simulink model "neww"  (R2023a)
settings: Solver=VariableStepAuto  StartTime=0.0  StopTime=0.5  RelTol=1e-3
libraries: spsMosfetLib x14, spsSeriesRLCBranchLib x13, simulink x6, spsDiodeLib x6, spsCurrentMeasurementLib x4, spsVoltageMeasurementLib x4, spsDCVoltageSourceLib x1, slpidlib x1, spsPVArrayLib x1, spsPWMGeneratorDCDCLib x1, spspowerguiLib x1
settings Model: Creator=91790  LastModifiedBy=USER
settings DataIOCC: ReturnWorkspaceOutputs=off
settings RTWCC: GPUComputeCapability=5.0

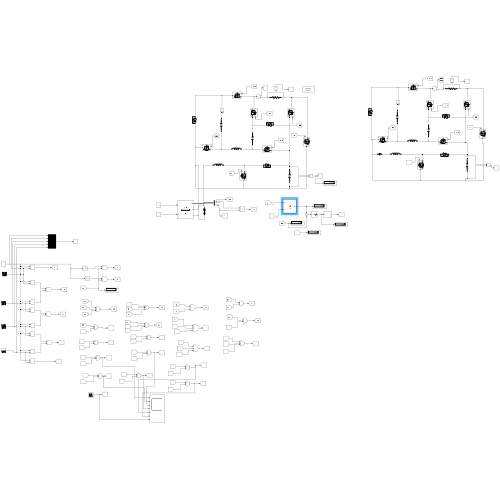
[thumbnail: Simulink's stored preview of the top-level diagram]
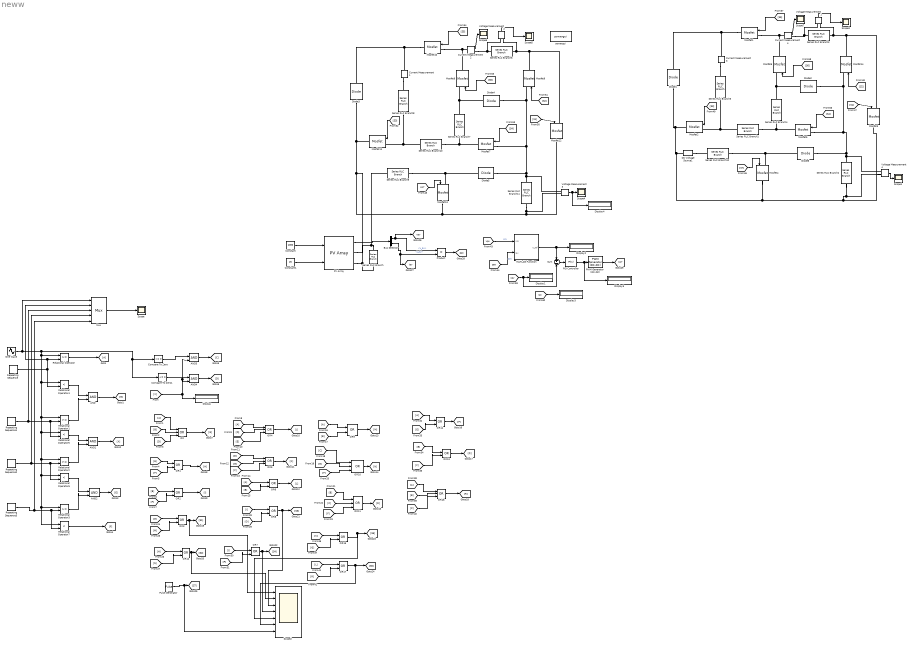
== system neww ==
  AND{,1..4} (5 alike) : Logic  IconShape=distinctive  AllPortsSameDT=off  OutDataTypeStr=boolean
  Bus Selector : BusSelector  OutputSignals=V_PV,I_PV
  Compare To Zero : simulink/Logic and Bit Operations/Compare To Zero  relop=>=  OutDataTypeStr=boolean
  Compare To Zero1 : simulink/Logic and Bit Operations/Compare To Zero  relop=<=  OutDataTypeStr=boolean
  Constant : Constant  Value=1000
  Constant1 : Constant  Value=25
  Current Measurement{1..4} (4 alike) : spsCurrentMeasurementLib/Current Measurement  PhasorSimulation=off  OutputType=Complex  PSBequivalent=0
  DC Voltage Source1 : spsDCVoltageSourceLib/DC Voltage Source  Amplitude=8  Measurements=None
  Diode{1..6} (6 alike) : spsDiodeLib/Diode  Ron=0.001  Lon=0  Vf=0.8  IC=0  UseSnubber=0  Rs=500  Cs=250e-9  Measurements=off
  Display{,1..5} (6 alike) : Display
  From{1,8,14,16,32,38} (6 alike) : From
  Goto : Goto
  MATLAB Function : MATLAB Function  TreatAsAtomicUnit=on  SystemSampleTime=1e-4
  Mosfet{1..14} (14 alike) : spsMosfetLib/Mosfet  Ron=0.1  Lon=0  Rd=0.01  Vfd=0  IC=0  Rs=1e5  Cs=inf  Measurements=off
  Mux : Mux  Inputs=5
  OR{,4..5,10..11,16} (6 alike) : Logic  Operator=OR  Inputs=3  IconShape=distinctive  AllPortsSameDT=off  OutDataTypeStr=boolean
  OR{1..3,6..9,12..15,17} (12 alike) : Logic  Operator=OR  IconShape=distinctive  AllPortsSameDT=off  OutDataTypeStr=boolean
  PID Controller : slpidlib/PID Controller  Controller=PI  Form=Parallel  TimeDomain=Continuous-time  UseExternalTs=off  SampleTime=-1  IntegratorMethod=Forward Euler  FilterMethod=Forward Euler  ControllerParametersSource=internal  P=0  I=-15  UseKiTs=off  D=0  N=100  UseFilter=on  TunerSelectOption=Transfer Function Based (PID Tuner App)  InitialConditionSource=internal  InitialConditionForIntegrator=0.5  InitialConditionForFilter=0  DifferentiatorICPrevScaledInput=0  ExternalReset=none  TrackingMode=off  Kt=1  LimitOutput=on  SatLimitsSource=internal  UpperSaturationLimit=0.95  LowerSaturationLimit=0.05  LinearizeAsGain=off  AntiWindupMode=none  Kb=1  LimitIntegrator=off  UpperIntegratorSaturationLimit=inf  LowerIntegratorSaturationLimit=-inf  POutMin=[]  POutMax=[]  IOutMin=[]  IOutMax=[]  DOutMin=[]  DOutMax=[]  NOutMin=[]  NOutMax=[]  SumOutMin=[]  SumOutMax=[]  SaturationOutMin=[]  SaturationOutMax=[]  PParamMin=[]  PParamMax=[]  IParamMin=[]  IParamMax=[]  DParamMin=[]  DParamMax=[]  NParamMin=[]  NParamMax=[]  KbParamMin=[]  KbParamMax=[]  KtParamMin=[]  KtParamMax=[]  KbOutMin=[]  KbOutMax=[]  KtOutMin=[]  KtOutMax=[]  IntegratorOutMin=[]  IntegratorOutMax=[]  FilterOutMin=[]  FilterOutMax=[]  SumI1OutMin=[]  SumI1OutMax=[]  SumI2OutMin=[]  SumI2OutMax=[]  SumI3OutMin=[]  SumI3OutMax=[]  SumI4OutMin=[]  SumI4OutMax=[]  SumDOutMin=[]  SumDOutMax=[]  DifferentiatorOutMin=[]  DifferentiatorOutMax=[]  FilterDiffOutCoefMin=[]  FilterDiffOutCoefMax=[]  ReciprocalOutMin=[]  ReciprocalOutMax=[]  SumDenOutMin=[]  SumDenOutMax=[]  SumNumOutMin=[]  SumNumOutMax=[]  DivideOutMin=[]  DivideOutMax=[]  UdiffTsProdOutMin=[]  UdiffTsProdOutMax=[]  NTsProdOutMin=[]  NTsProdOutMax=[]  UintegralTsProdOutMin=[]  UintegralTsProdOutMax=[]  UngainTsProdOutMin=[]  UngainTsProdOutMax=[]  ClampingZeroOutDataTypeStr=Inherit: Inherit via back propagation  ClampingZeroOutMin=[]  ClampingZeroOutMax=[]  FilterDenConstantOutDataTypeStr=Inherit: Inherit via back propagation  FilterDenConstantOutMin=[]  FilterDenConstantOutMax=[]  PCopyOutDataTypeStr=Inherit: Inherit via back propagation  PCopyOutMin=[]  PCopyOutMax=[]  NCopyOutDataTypeStr=Inherit: Inherit via back propagation  NCopyOutMin=[]  NCopyOutMax=[]  IntegratorContinuousStateAttributes=''  IntegratorStateMustResolveToSignalObject=off  IntegratorRTWStateStorageClass=Auto  FilterContinuousStateAttributes=''  FilterStateMustResolveToSignalObject=off  FilterRTWStateStorageClass=Auto  ParallelPVariant=InternalParameters  IdealPVariant=Disabled  IVariant=InternalParameters  DVariant=Disabled  IntegratorVariant=Continuous  SatVariant=Enabled  AWVariant=Passthrough  PCopyVariant=Disabled  TRVariant=Disabled  FdbkBlocksVariant=Forward  IdealPFdbkVariant=Disabled  SatFdbkVariant=Disabled  DerivativeFilterVariant=Disabled  NVariant=Disabled  NCopyVariant=Disabled_SignalSpec  FilterICVariant=Disabled  IntegratorICVariant=InternalICs  ExternalResetVariant=Disabled  TRSumVariant=Passthrough  SumFdbkVariant=Disabled  SumVariant=Sum_PI  TsampFilterVariant=InternalTs  TsampNgainVariant=Passthrough  TsampIntegralVariant=Disabled_SignalSpec  ExternalSaturationOutDataTypeStr=Inherit: Same as second input
  PV Array : spsPVArrayLib/PV Array  Npar=1  Nser=1  PlotType=array @ 1000 W/m2 & specified temperatures  S_vec="[ 1000  500  100 ]"  Temp_C_vec="[ 45 25  ]"  ModuleName=User-defined  PlotWhenSelected=off  Pm=74.8334  Ncell=36  Voc=21.89  Isc=4.48  Vm=17.86  Im=4.19  beta_Voc_pc=-0.36099  alpha_Isc_pc=0.102  beta_Voc=-0.079021  alpha_Isc=0.0045696  IL=4.485  I0=1.6678e-10  nI=0.98621  Rsh=286.612  Rs=0.317  RobustModel=off  RobustCellTemperature=313.3991  BAL=on  Tc=1e-6  Tfilter=5e-5
  PWM Generator (DC-DC) : spsPWMGeneratorDCDCLib/PWM Generator (DC-DC)  Fsw=2500  Ts=0
  Product : Product
  Pulse Generator : DiscretePulseGenerator  PulseType=Time based  Period=1/21000  PulseWidth=75
  Relational Operator{,1..3} (4 alike) : RelationalOperator  OutDataTypeStr=boolean  RndMeth=Simplest  InputSameDT=off
  Relational Operator{4..7} (4 alike) : RelationalOperator  Operator=<  OutDataTypeStr=boolean  RndMeth=Simplest  InputSameDT=off
  Repeating Sequence : simulink/Sources/Repeating Sequence  rep_seq_t=[0 1/4 1/2]/2500  rep_seq_y=[1 0.5 1]
  Repeating Sequence1 : simulink/Sources/Repeating Sequence  rep_seq_t=[0 1/4 1/2]/2500  rep_seq_y=[0.5 0 0.5]
  Repeating Sequence2 : simulink/Sources/Repeating Sequence  rep_seq_t=[0 1/4 1/2]/2500  rep_seq_y=[0 -0.5 0]
  Repeating Sequence3 : simulink/Sources/Repeating Sequence  rep_seq_t=[0 1/4 1/2]/2500  rep_seq_y=[-0.5 -1 -0.5]
  Scope{,1,3..7} (7 alike) : Scope
  Scope2 : Scope  NumInputPorts=7
  Series RLC Branch : spsSeriesRLCBranchLib/Series RLC Branch  LConnTagsString=__new0  RConnTagsString=__new0  BranchType=RC  Resistance=0.11e-4  Inductance=1e-3  SetiL0=off  InitialCurrent=0  Capacitance=1000e-6  Setx0=off  InitialVoltage=0  Measurements=None
  Series RLC Branch1 : spsSeriesRLCBranchLib/Series RLC Branch  LConnTagsString=__new0  RConnTagsString=__new0  BranchType=L  Resistance=100  Inductance=1e-3  SetiL0=off  InitialCurrent=0  Capacitance=1e-6  Setx0=off  InitialVoltage=0  Measurements=Branch voltage and current
  Series RLC Branch10 : spsSeriesRLCBranchLib/Series RLC Branch  LConnTagsString=__new0  RConnTagsString=__new0  BranchType=L  Resistance=100  Inductance=1e-3  SetiL0=off  InitialCurrent=0  Capacitance=1e-6  Setx0=off  InitialVoltage=0  Measurements=Branch voltage and current
  Series RLC Branch11 : spsSeriesRLCBranchLib/Series RLC Branch  LConnTagsString=__new0  RConnTagsString=__new0  BranchType=C  Resistance=100  Inductance=1e-3  SetiL0=off  InitialCurrent=0  Capacitance=4700e-6  Setx0=off  InitialVoltage=0  Measurements=None
  Series RLC Branch12 : spsSeriesRLCBranchLib/Series RLC Branch  LConnTagsString=__new0  RConnTagsString=__new0  BranchType=L  Resistance=100  Inductance=1e-3  SetiL0=off  InitialCurrent=0  Capacitance=1e-6  Setx0=off  InitialVoltage=0  Measurements=None
  Series RLC Branch{2,4..5,7..8} (5 alike) : spsSeriesRLCBranchLib/Series RLC Branch  LConnTagsString=__new0  RConnTagsString=__new0  BranchType=C  Resistance=100  Inductance=1e-3  SetiL0=off  InitialCurrent=0  Capacitance=2200e-6  Setx0=off  InitialVoltage=0  Measurements=None
  Series RLC Branch3 : spsSeriesRLCBranchLib/Series RLC Branch  LConnTagsString=__new0  RConnTagsString=__new0  BranchType=R  Resistance=100  Inductance=5e-3  SetiL0=off  InitialCurrent=0  Capacitance=1e-6  Setx0=off  InitialVoltage=0  Measurements=None
  Series RLC Branch6 : spsSeriesRLCBranchLib/Series RLC Branch  LConnTagsString=__new0  RConnTagsString=__new0  BranchType=R  Resistance=100  Inductance=5e-3  SetiL0=off  InitialCurrent=0  Capacitance=1e-6  Setx0=off  InitialVoltage=0  Measurements=None
  Series RLC Branch9 : spsSeriesRLCBranchLib/Series RLC Branch  LConnTagsString=__new0  RConnTagsString=__new0  BranchType=L  Resistance=100  Inductance=1e-3  SetiL0=off  InitialCurrent=0  Capacitance=1e-6  Setx0=off  InitialVoltage=0  Measurements=None
  Sine Wave : Sin  Amplitude=0.98  Frequency=2*pi*50  SampleTime=0
  Sum : Sum  Inputs=+-
  Voltage Measurement{1..4} (4 alike) : spsVoltageMeasurementLib/Voltage Measurement  PhasorSimulation=off  OutputType=Complex  PSBequivalent=0
  powergui : spspowerguiLib/powergui  Priority=1  SimulationMode=Discrete  SampleTime=5e-6  frequency=60  Iterations=50  frequencyindice=0  Pbase=100e6  ErrMax=1e-4  UnitsV=kV  UnitsW=MW  buscounter=0  FunctionMessages=off  echomessages=off  EnableUseOfTLC=off  CurrentSourceSwitches=off  DisableSnubberDevices=off  DisableRonSwitches=off  DisableVfSwitches=off  DisplayEquations=off  AutomaticDiscreteSolvers=off  SolverType=Tustin/Backward Euler (TBE)  Interpol=off  ExternalGateDelay=off  methode=off  Ts=100  x0status=blocks  SPID=on  SwTol=0  HookPort=off  NonlinearTolerance=1e-4  nMaxIteration=100  ContinueOnMaxIteration=off  RestoreLinks=warning  ResistiveCurrentMeasurement=off  Frange=[0:2:500]  Ylog=off  Xlog=on  ShowGrid=off  save=off  variable=ZData  structure=0  ZoomFFT=off  StartTime=0.0  cycles=1  DisplayStyle=1  fundamental=60  FreqAxis=off  MaxFrequency=1000  frequencyindicesteady=1  RmsSteady=1  display=off
  tag scope: ipv=global, ppv=global, ss7=global, vpv=global
  wires:
  Repeating Sequence/1 -> Relational Operator4/2, Mux/2, Relational Operator/2
  Repeating Sequence1/1 -> Relational Operator5/2, Relational Operator1/2, Mux/3
  Repeating Sequence2/1 -> Relational Operator2/2, Relational Operator6/2, Mux/4
  Repeating Sequence3/1 -> Relational Operator3/2, Relational Operator7/2, Mux/5
  Relational Operator4/1 -> AND/1
  Relational Operator1/1 -> AND/2
  Relational Operator5/1 -> AND1/1
  Relational Operator2/1 -> AND1/2
  Relational Operator6/1 -> AND2/1
  Relational Operator3/1 -> AND2/2
  Compare To Zero/1 -> AND3/1
  Compare To Zero1/1 -> AND4/1
  [X] -> AND4/2, AND3/2, Display/1
  AND3/1 -> [C]
  AND4/1 -> [D]
  From1/1 -> OR/1
  [B] -> OR/2
  [D] -> OR/3
  [E] -> OR1/1
  [F] -> OR1/2
  [B] -> OR2/1
  [F] -> OR2/2
  OR/1 -> [G]
  OR1/1 -> [H]
  OR2/1 -> [I]
  OR4/1 -> [J]
  From8/1 -> OR4/1
  [D] -> OR4/2
  [E] -> OR4/3
  [D] -> OR5/1
  [E] -> OR5/2
  [F] -> OR5/3
  From14/1 -> OR6/1
  [B] -> OR6/2
  OR5/1 -> [K]
  OR6/1 -> [L]
  OR9/1 -> [M]
  [C] -> OR10/1
  [F] -> OR10/3
  [F] -> OR11/3
  OR10/1 -> [N]
  [E] -> OR10/2
  OR11/1 -> [O]
  [C] -> OR11/2
  [B] -> OR11/1
  [G] -> OR3/1
  [M] -> OR3/2
  [N] -> OR12/2
  [H] -> OR12/1
  [J] -> OR7/1
  [P] -> OR7/2
  [O] -> OR8/2
  [I] -> OR8/1
  [F] -> OR13/2
  [E] -> OR14/2
  From32/1 -> OR14/1
  [E] -> OR13/1
  OR13/1 -> [Q]
  OR14/1 -> [P]
  [Q] -> OR15/2
  [K] -> OR15/1
  From38/1 -> OR16/1
  OR16/1 -> [R]
  [B] -> OR16/2
  [C] -> OR16/3
  Relational Operator/1 -> Goto/1
  AND/1 -> [B]
  AND1/1 -> [X]
  AND2/1 -> [E]
  Relational Operator7/1 -> [F]
  Sine Wave/1 -> Mux/1, Compare To Zero1/1, Compare To Zero/1, Relational Operator/1, Relational Operator4/1, Relational Operator1/1, Relational Operator5/1, Relational Operator2/1, Relational Operator6/1, Relational Operator3/1, Relational Operator7/1
  Mux/1 -> Scope/1
  OR3/1 -> Scope2/1, [S1]
  OR12/1 -> Scope2/2, [S2]
  OR8/1 -> Scope2/3, [S3]
  OR7/1 -> Scope2/4, [S4]
  [L] -> OR17/1
  [R] -> OR17/2
  OR15/1 -> Scope2/5, [S5]
  OR17/1 -> Scope2/6, [S6]
  Pulse Generator/1 -> Scope2/7, [S7]
  From16/1 -> OR9/1
  [B] -> OR9/2
  Voltage Measurement3/1 -> Display4/1, Scope4/1
  [ss7] -> Mosfet13/1
  Voltage Measurement2/1 -> Scope5/1
  [S2] -> Mosfet9/1
  [S1] -> Mosfet12/1
  [S6] -> Mosfet8/1
  [S5] -> Mosfet10/1
  [S4] -> Mosfet7/1
  [S3] -> Mosfet11/1
  Current Measurement2/1 -> Scope6/1
  Constant1/1 -> PV Array/2
  Constant/1 -> PV Array/1
  Bus Selector/2 -> [ipv], Product/2  "<I_PV>"
  Bus Selector/1 -> Product/1, [vpv]  "<V_PV>"
  PV Array/1 -> Bus Selector/1
  [ppv] -> MATLAB Function/2(ipv)  "ppv"
  Product/1 -> [ppv]
  [vpv] -> MATLAB Function/1(vpv)  "vpv"
  MATLAB Function/1(V_ref) -> Sum/1, Display2/1
  Current Measurement4/1 -> Scope7/1
  [S3] -> Mosfet2/1
  [S4] -> Mosfet5/1
  [S5] -> Mosfet1/1
  [S6] -> Mosfet6/1
  [S1] -> Mosfet3/1
  [S2] -> Mosfet14/1
  Voltage Measurement1/1 -> Scope3/1
  [S7] -> Mosfet4/1
  Voltage Measurement4/1 -> Scope1/1
  [vpv] -> Sum/2, Display1/1
  [ipv] -> Display3/1
  Sum/1 -> PID Controller/1
  PID Controller/1 -> Display5/1, PWM Generator (DC-DC)/1
  PWM Generator (DC-DC)/1 -> [ss7]
  connections:
  Diode3/RConn1 -- Mosfet13/RConn1 -- Series RLC Branch11/RConn1 -- Voltage Measurement3/LConn2 -- Mosfet12/RConn1 -- PV Array/RConn2 -- Series RLC Branch/RConn1 -- Mosfet11/RConn1
  Voltage Measurement2/LConn1 -- Series RLC Branch6/RConn1 -- Mosfet12/LConn1 -- Mosfet9/RConn1
  Mosfet10/RConn1 -- Diode3/LConn1 -- Current Measurement1/LConn1
  Mosfet10/LConn1 -- Current Measurement2/LConn1 -- Mosfet8/RConn1
  Mosfet11/LConn1 -- Series RLC Branch8/LConn1 -- Series RLC Branch10/LConn1
  Diode4/LConn1 -- Mosfet7/LConn1 -- Voltage Measurement3/LConn1 -- Series RLC Branch11/LConn1 -- Diode5/RConn1 -- Mosfet9/LConn1
  Series RLC Branch7/RConn1 -- Mosfet7/RConn1 -- Series RLC Branch10/RConn1
  Diode4/RConn1 -- Series RLC Branch7/LConn1 -- Mosfet8/LConn1
  Series RLC Branch9/RConn1 -- Mosfet13/LConn1 -- Diode5/LConn1
  Current Measurement1/RConn1 -- Series RLC Branch8/RConn1
  Series RLC Branch6/LConn1 -- Voltage Measurement2/LConn2 -- Current Measurement2/RConn1
  Mosfet3/RConn1 -- Voltage Measurement4/LConn2 -- Series RLC Branch2/RConn1 -- Diode1/RConn1 -- Mosfet2/RConn1 -- DC Voltage Source1/LConn1 -- Mosfet4/RConn1
  Voltage Measurement1/LConn1 -- Mosfet14/RConn1 -- Mosfet3/LConn1 -- Series RLC Branch3/RConn1
  Mosfet1/RConn1 -- Current Measurement3/LConn1 -- Diode1/LConn1
  Mosfet1/LConn1 -- Mosfet6/RConn1 -- Current Measurement4/LConn1
  Mosfet2/LConn1 -- Series RLC Branch1/LConn1 -- Series RLC Branch5/LConn1
  Diode2/LConn1 -- Mosfet14/LConn1 -- Diode6/RConn1 -- Series RLC Branch2/LConn1 -- Voltage Measurement4/LConn1 -- Mosfet5/LConn1
  Series RLC Branch4/RConn1 -- Series RLC Branch1/RConn1 -- Mosfet5/RConn1
  Diode2/RConn1 -- Mosfet6/LConn1 -- Series RLC Branch4/LConn1
  Series RLC Branch12/RConn1 -- Diode6/LConn1 -- Mosfet4/LConn1
  Series RLC Branch3/LConn1 -- Current Measurement4/RConn1 -- Voltage Measurement1/LConn2
  Current Measurement3/RConn1 -- Series RLC Branch5/RConn1
  DC Voltage Source1/RConn1 -- Series RLC Branch12/LConn1
  Series RLC Branch/LConn1 -- PV Array/RConn1 -- Series RLC Branch9/LConn1

== matlab function neww/MATLAB Function ==
  data: vpv input; V_ref output; ipv input
function V_ref = IC_Vref(vpv, ipv)
% Incremental Conductance (IC) MPPT Algorithm for V_ref control
%
% This function determines the new reference voltage (V_ref) for the PV
% system based on the Incremental Conductance rule: dI/dV = -I/V at MPP.
%
% Inputs:
%   vpv - Current PV Voltage (V)
%   ipv - Current PV Current (I)
%
% Output:
%   V_ref - New reference voltage (V_ref)

% --- Persistent variables to remember state between calls ---
persistent v_pre i_pre V_ref_pre;
% --- Define Panel Limits and Step Size ---
persistent V_ref_max V_ref_min del_V;

% --- Step size for voltage perturbation ---
del_V = 0.05; % Perturb by a small voltage step (e.g., 0.05 Volts)

% --- Initialization (runs only once) ---
if isempty(V_ref_pre)
    % Initial values based on your panel's datasheet (Vmp)
    v_pre = 17.19;     
    i_pre = 74 / 17.19; % Initial current estimate
    V_ref_pre = 17.19; % Start at Vmp
    
    % --- SET LIMITS HERE ---
    V_ref_max = 21.19; % Open Circuit Voltage (Voc)
    V_ref_min = 5.0;   % A safe minimum limit
end

% --- Calculate Changes (Increments) ---
Delta_V = vpv - v_pre;
Delta_I = ipv - i_pre;

% --- Core IC Decision Logic ---
V_ref = V_ref_pre; % Initialize V_ref to the previous value (No change)

% Case 1: Change in Voltage is ZERO (Delta_V = 0)
% This happens if the system is holding steady or if the PI controller is very stiff.
if (Delta_V == 0)
    % Check if power is increasing (I increases) or decreasing (I decreases)
    if (Delta_I > 0)
        % V is constant, I is increasing -> Still increasing power, continue
        V_ref = V_ref_pre + del_V;
    elseif (Delta_I < 0)
        % V is constant, I is decreasing -> Power dropping, reverse
        V_ref = V_ref_pre - del_V;
    else
        % Power is stable, hold steady
        V_ref = V_ref_pre;
    end

% Case 2: Change in Voltage is NON-ZERO (Delta_V != 0)
else
    % Calculate Incremental Conductance (dI/dV)
    Inc_Cond = Delta_I / Delta_V; 
    
    % Calculate Negative Instantaneous Conductance (-I/V)
    Inst_Cond_Neg = -ipv / vpv; 

    % --- INC RULES ---
    
    if (Inc_Cond == Inst_Cond_Neg) % Condition 1: At MPP (dI/dV = -I/V)
        % Hold steady at the current V_ref
        V_ref = V_ref_pre;
        
    elseif (Inc_Cond > Inst_Cond_Neg) % Condition 2: Left of MPP (V is too LOW)
        % We need to increase V, so decrease V_ref
        % The sign of the perturbation depends on the prior direction
        if (Delta_V > 0)
            V_ref = V_ref_pre + del_V; % V increased, was good, continue
        else
            V_ref = V_ref_pre - del_V; % V decreased, was bad, reverse
        end
        
    elseif (Inc_Cond < Inst_Cond_Neg) % Condition 3: Right of MPP (V is too HIGH)
        % We need to decrease V, so decrease V_ref
        % The sign of the perturbation depends on the prior direction
        if (Delta_V < 0)
            V_ref = V_ref_pre - del_V; % V decreased, was good, continue
        else
            V_ref = V_ref_pre + del_V; % V increased, was bad, reverse
        end
    end
end

% --- Apply V_ref Limits ---
if V_ref > V_ref_max
    V_ref = V_ref_max; % Don't go above Voc
end
if V_ref < V_ref_min
    V_ref = V_ref_min; % Don't go below the minimum
end

% --- Update persistent variables for the next run ---
V_ref_pre = V_ref;
v_pre = vpv;
i_pre = ipv;

end
